simulink model "Grundregler_ENG"  (R2018b)
settings: Solver=VariableStepAuto  StartTime=0.0  StopTime=10.0  RelTol=1e-3
settings Model: Creator=F58925B  LastModifiedBy=F58925B

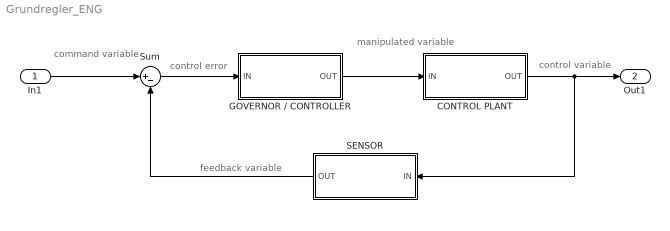
== system Grundregler_ENG ==
  note: control variable
  note: manipulated
      |    variable
  note: control error
  note: command variable
  note: feedback variable
  In1 : Inport
  CONTROL PLANT : Subsystem
  GOVERNOR / CONTROLLER : Subsystem
  SENSOR : Subsystem
  Sum : Sum  Inputs=|+-
  Out1 : Outport  Port=2
  wires:
  CONTROL PLANT/1(OUT) -> Out1/1, SENSOR/1(IN)
  GOVERNOR / CONTROLLER/1(OUT) -> CONTROL PLANT/1(IN)
  Sum/1 -> GOVERNOR / CONTROLLER/1(IN)
  In1/1 -> Sum/1
  SENSOR/1(OUT) -> Sum/2

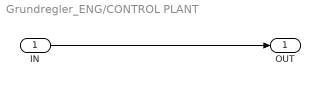
== system Grundregler_ENG/CONTROL PLANT ==
  IN : Inport
  OUT : Outport
  wires:
  IN/1 -> OUT/1

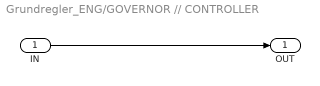
== system Grundregler_ENG/GOVERNOR // CONTROLLER ==
  IN : Inport
  OUT : Outport
  wires:
  IN/1 -> OUT/1

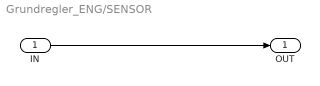
== system Grundregler_ENG/SENSOR ==
  IN : Inport
  OUT : Outport
  wires:
  IN/1 -> OUT/1
